simulink model "sampleModel1767_4_sub_sub_sub"  (R2023a)
settings: Solver=VariableStepAuto  StartTime=0.0  StopTime=10.0  RelTol=1e-3
libraries: simulink x5, hdlsllib x3
settings Model: Creator=user1  LastModifiedBy=user1

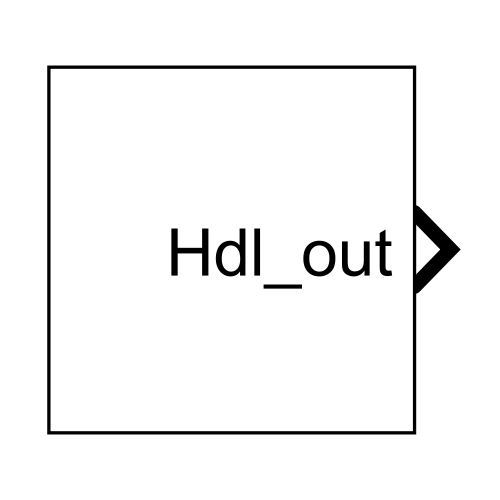
[thumbnail: Simulink's stored preview of the top-level diagram]
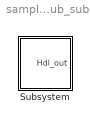
== system sampleModel1767_4_sub_sub_sub ==
  Subsystem : Subsystem

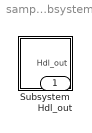
== system sampleModel1767_4_sub_sub_sub/Subsystem ==
  Subsystem : Subsystem
  Hdl_out : Outport  OutDataTypeStr=uint8

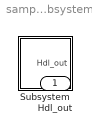
== system sampleModel1767_4_sub_sub_sub/Subsystem/Subsystem ==
  Subsystem : Subsystem
  Hdl_out : Outport  OutDataTypeStr=uint8

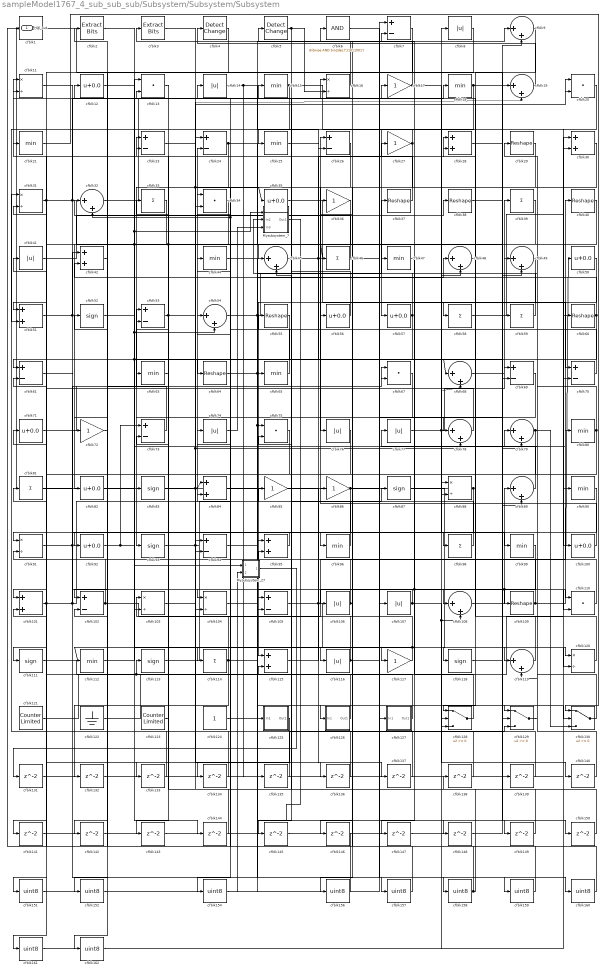
== system sampleModel1767_4_sub_sub_sub/Subsystem/Subsystem/Subsystem ==
  Mysubsystem_27 : Subsystem  TreatAsAtomicUnit=on  RTWFcnName=Mysubsystem_27
      settings: RTWFcnNameOpts=User specified  RTWFileNameOpts=Use function name
  Mysubsystem_7 : Subsystem  TreatAsAtomicUnit=on  RTWFcnName=Mysubsystem_7
      settings: RTWFcnNameOpts=User specified  RTWFileNameOpts=Use function name
  cfblk1 : hdlsllib/Logic and Bit Operations/Compare To Constant  relop=<=  const=3.0  OutDataTypeStr=uint8
  cfblk{12,35,50,56..57,71,82,92,100} (9 alike) : Bias  Bias=0.0  SaturateOnIntegerOverflow=off
  cfblk{28,30,42,51,84,95,101,115} (8 alike) : Sum  OutDataTypeStr=uint8
  cfblk{7,23..24,26,53,61,69..70,73,94,102,105} (12 alike) : Sum  Inputs=+-  OutDataTypeStr=uint8
  cfblk{11,16,31,88,91,103..104,120} (8 alike) : Product  Inputs=*/  OutDataTypeStr=uint8  RndMeth=Zero  SaturateOnIntegerOverflow=on
  cfblk{8,14,41,74,76..77,106..107,116} (9 alike) : Abs  OutDataTypeStr=uint8  SaturateOnIntegerOverflow=off
  cfblk{9,19,32,45,48..49,54,68,78..79,89,108,119} (13 alike) : Sum  Inputs=|++  OutDataTypeStr=uint8
  cfblk{29,37..38,40,55,60,64,109} (8 alike) : Reshape
  cfblk{13,20,34,67,75,110} (6 alike) : DotProduct  OutDataTypeStr=uint8
  cfblk{52,83,87,93,111,113,118} (7 alike) : Signum
  cfblk{15,18,21,25,44,47,63,65,80,90,96,99,112} (13 alike) : MinMax  OutDataTypeStr=uint8
  cfblk{33,39,46,58..59,81,98,114} (8 alike) : Sum  Inputs=+  OutDataTypeStr=uint8
  cfblk{17,27,36,72,85..86,117} (7 alike) : Gain  OutDataTypeStr=uint8
  cfblk121 : hdlsllib/Sources/Counter Limited  uplimit=7  tsamp=-1
  cfblk122 : Ground
  cfblk123 : hdlsllib/Sources/Counter Limited  uplimit=7  tsamp=-1
  cfblk124 : Constant  OutDataTypeStr=uint8  SampleTime=-1
  cfblk125 : Subsystem
      settings: LibrarySourceBlock=|
      | hdlsllib/Ports &
      | Subsystems/Subsystem
  cfblk126 : Subsystem
      settings: LibrarySourceBlock=|
      | hdlsllib/Ports &
      | Subsystems/Subsystem
  cfblk127 : Subsystem
      settings: LibrarySourceBlock=|
      | hdlsllib/Ports &
      | Subsystems/Subsystem
  cfblk128 : Switch  OutDataTypeStr=uint8  SaturateOnIntegerOverflow=off  InputSameDT=off
  cfblk129 : Switch  OutDataTypeStr=uint8  SaturateOnIntegerOverflow=off  InputSameDT=off
  cfblk130 : Switch  OutDataTypeStr=uint8  SaturateOnIntegerOverflow=off  InputSameDT=off
  cfblk{131..150} (20 alike) : Delay  SampleTime=1
  cfblk{151..152,154,156..162} (10 alike) : DataTypeConversion  OutDataTypeStr=uint8  SaturateOnIntegerOverflow=off  RndMeth=Floor
  cfblk2 : simulink/Logic and Bit Operations/Extract Bits  bitsToExtract=Upper half  numBits=8  bitIdxRange=[0 7]  outScalingMode=Preserve fixed-point scaling
      settings: LibrarySourceBlock=|
      | hdlsllib/Logic and Bit
      | Operations/Extract Bits
  cfblk3 : simulink/Logic and Bit Operations/Extract Bits  bitsToExtract=Upper half  numBits=8  bitIdxRange=[0 7]  outScalingMode=Preserve fixed-point scaling
      settings: LibrarySourceBlock=|
      | hdlsllib/Logic and Bit
      | Operations/Extract Bits
  cfblk4 : simulink/Logic and Bit Operations/Detect Change  vinit=0  OutDataTypeStr=uint8
      settings: LibrarySourceBlock=|
      | hdlsllib/Logic and Bit
      | Operations/Detect
      | Change
  cfblk5 : simulink/Logic and Bit Operations/Detect Change  vinit=0  OutDataTypeStr=uint8
      settings: LibrarySourceBlock=|
      | hdlsllib/Logic and Bit
      | Operations/Detect
      | Change
  cfblk6 : simulink/Logic and Bit Operations/Bitwise Operator  logicop=AND  UseBitMask=on  BitMask=bin2dec('11011001')  BitMaskRealWorld=Stored Integer
      settings: LibrarySourceBlock=|
      | hdlsllib/Logic and Bit
      | Operations/Bitwise
      | Operator
  Hdl_out : Outport  OutDataTypeStr=uint8
  wires:
  cfblk32/1 -> cfblk14/1
  cfblk31/1 -> cfblk61/1, cfblk18/1, cfblk45/1
  cfblk99/1 -> cfblk147/1, cfblk146/1
  cfblk33/1 -> cfblk82/1
  cfblk101/1 -> cfblk41/1, cfblk67/1, cfblk24/2
  cfblk65/1 -> cfblk34/1
  cfblk67/1 -> cfblk93/1
  cfblk21/1 -> cfblk130/1
  cfblk7/1 -> cfblk102/1
  cfblk102/1 -> cfblk71/1, cfblk40/1
  cfblk41/1 -> cfblk38/1
  cfblk119/1 -> cfblk12/1
  cfblk109/1 -> cfblk31/2, cfblk50/1
  cfblk108/1 -> cfblk89/1
  cfblk73/1 -> cfblk52/1
  cfblk55/1 -> cfblk115/1
  cfblk92/1 -> cfblk73/1, cfblk80/1
  cfblk6/1 -> cfblk158/1
  cfblk59/1 -> cfblk15/1
  cfblk29/1 -> cfblk83/1
  cfblk9/1 -> cfblk128/1
  cfblk11/1 -> cfblk96/1
  cfblk49/1 -> cfblk65/1
  cfblk80/1 -> cfblk49/1, cfblk91/1
  cfblk98/1 -> cfblk26/1
  cfblk71/1 -> cfblk53/1
  cfblk19/1 -> cfblk4/1
  cfblk68/1 -> cfblk39/1
  cfblk57/1 -> cfblk111/1, Mysubsystem_7/2(In2)
  cfblk40/1 -> cfblk76/1
  cfblk30/1 -> cfblk56/1
  cfblk113/1 -> cfblk85/1
  cfblk17/1 -> cfblk79/2, cfblk5/1
  cfblk34/1 -> cfblk143/1, cfblk72/1
  cfblk111/1 -> cfblk115/2
  cfblk95/1 -> cfblk92/1
  cfblk112/1 -> cfblk13/1
  cfblk46/1 -> cfblk78/1, cfblk32/1
  cfblk18/1 -> cfblk89/2, cfblk57/1
  cfblk93/1 -> cfblk110/1, cfblk19/2, cfblk87/1
  cfblk87/1 -> cfblk120/1
  cfblk122/1 -> cfblk8/1
  cfblk100/1 -> cfblk86/1
  cfblk86/1 -> cfblk103/2, cfblk129/1
  cfblk35/1 -> cfblk70/1
  cfblk79/1 -> cfblk130/3, cfblk95/1
  cfblk47/1 -> cfblk117/1
  cfblk61/1 -> cfblk98/1
  cfblk27/1 -> cfblk25/1, cfblk116/1
  cfblk54/1 -> cfblk130/2, cfblk48/1, cfblk37/1
  cfblk106/1 -> cfblk156/1, cfblk55/1
  cfblk45/1 -> cfblk27/1, cfblk88/2
  cfblk83/1 -> cfblk84/1, cfblk20/1, cfblk78/2
  cfblk39/1 -> cfblk64/1
  cfblk64/1 -> cfblk148/1, cfblk47/1
  cfblk115/1 -> cfblk28/1
  cfblk128/1 -> cfblk7/2
  cfblk105/1 -> cfblk79/1, cfblk127/1(In1)
  cfblk126/1(Out1) -> cfblk61/2, cfblk113/1
  cfblk16/1 -> cfblk3/1
  cfblk89/1 -> cfblk17/1
  cfblk70/1 -> cfblk32/2, cfblk13/2
  cfblk15/1 -> cfblk51/2, cfblk100/1
  cfblk37/1 -> cfblk11/1
  cfblk77/1 -> cfblk99/1, cfblk69/1
  cfblk84/1 -> cfblk110/2, cfblk109/1
  cfblk14/1 -> cfblk135/1, cfblk26/2
  cfblk50/1 -> cfblk58/1
  cfblk53/1 -> cfblk33/1, cfblk120/2
  cfblk118/1 -> cfblk19/1
  cfblk107/1 -> cfblk140/1, cfblk106/1
  cfblk120/1 -> cfblk28/2
  cfblk58/1 -> cfblk30/2
  cfblk94/1 -> cfblk9/1, cfblk75/1
  cfblk91/1 -> cfblk157/1, cfblk67/2
  cfblk48/1 -> cfblk108/1
  cfblk82/1 -> cfblk16/1, Mysubsystem_7/1(In1)
  cfblk5/1 -> cfblk16/2, cfblk105/1
  cfblk76/1 -> cfblk114/1
  cfblk90/1 -> cfblk161/1
  cfblk12/1 -> cfblk46/1, cfblk54/2, cfblk118/1, cfblk68/1
  cfblk110/1 -> cfblk36/1
  cfblk88/1 -> Hdl_out/1, cfblk101/1
  cfblk23/1 -> cfblk119/1, cfblk35/1
  cfblk121/1 -> cfblk60/1
  cfblk51/1 -> cfblk160/1, cfblk42/1
  cfblk114/1 -> cfblk132/1, cfblk20/2, cfblk23/2
  cfblk127/1(Out1) -> cfblk103/1
  cfblk123/1 -> cfblk23/1
  cfblk117/1 -> cfblk112/1, cfblk95/2
  cfblk20/1 -> cfblk70/2
  cfblk56/1 -> cfblk11/2
  cfblk24/1 -> cfblk49/2, cfblk94/2
  cfblk130/1 -> cfblk77/1
  cfblk81/1 -> cfblk104/1
  cfblk8/1 -> cfblk51/1
  cfblk78/1 -> cfblk21/1
  cfblk124/1 -> cfblk105/2
  cfblk25/1 -> cfblk69/2
  cfblk13/1 -> cfblk63/1
  cfblk129/1 -> cfblk29/1
  cfblk1/1 -> cfblk59/1
  cfblk60/1 -> cfblk42/2, cfblk104/2
  cfblk104/1 -> cfblk126/1(In1)
  cfblk96/1 -> cfblk75/2
  cfblk3/1 -> cfblk34/2
  cfblk116/1 -> cfblk73/2, cfblk128/3
  cfblk131/1 -> cfblk30/1
  cfblk132/1 -> cfblk94/1
  cfblk63/1 -> cfblk133/1
  cfblk133/1 -> cfblk31/1
  cfblk26/1 -> cfblk134/1
  cfblk134/1 -> cfblk101/2
  cfblk135/1 -> cfblk129/3
  cfblk103/1 -> cfblk136/1
  cfblk136/1 -> cfblk54/1
  cfblk85/1 -> cfblk137/1
  cfblk137/1 -> cfblk84/2
  cfblk138/1 -> cfblk91/2
  cfblk28/1 -> cfblk139/1
  cfblk139/1 -> cfblk88/1
  cfblk140/1 -> cfblk119/2
  cfblk36/1 -> cfblk141/1
  cfblk141/1 -> cfblk128/2
  cfblk72/1 -> cfblk142/1
  cfblk142/1 -> cfblk102/2
  cfblk143/1 -> cfblk9/2
  cfblk52/1 -> cfblk144/1
  cfblk144/1 -> cfblk24/1
  cfblk69/1 -> cfblk145/1
  cfblk145/1 -> cfblk7/1
  cfblk146/1 -> cfblk1/1
  cfblk147/1 -> cfblk48/2
  cfblk148/1 -> cfblk129/2
  cfblk149/1 -> cfblk53/2
  cfblk38/1 -> cfblk150/1
  cfblk150/1 -> cfblk45/2
  cfblk125/1(Out1) -> cfblk151/1
  cfblk151/1 -> cfblk107/1
  cfblk4/1 -> cfblk152/1
  cfblk152/1 -> cfblk125/1(In1)
  cfblk75/1 -> cfblk154/1
  cfblk156/1 -> cfblk2/1
  cfblk157/1 -> cfblk6/1
  cfblk158/1 -> cfblk81/1, cfblk138/1
  cfblk44/1 -> cfblk159/1
  cfblk159/1 -> cfblk74/1
  cfblk160/1 -> cfblk44/1
  cfblk161/1 -> cfblk108/2, cfblk68/2
  cfblk42/1 -> cfblk162/1
  cfblk162/1 -> cfblk90/1
  cfblk74/1 -> Mysubsystem_7/3(In3)
  Mysubsystem_7/1(Out1) -> cfblk149/1
  cfblk2/1 -> Mysubsystem_27/1(In1)
  cfblk154/1 -> Mysubsystem_27/2(In2)
  Mysubsystem_27/1(Out1) -> cfblk131/1

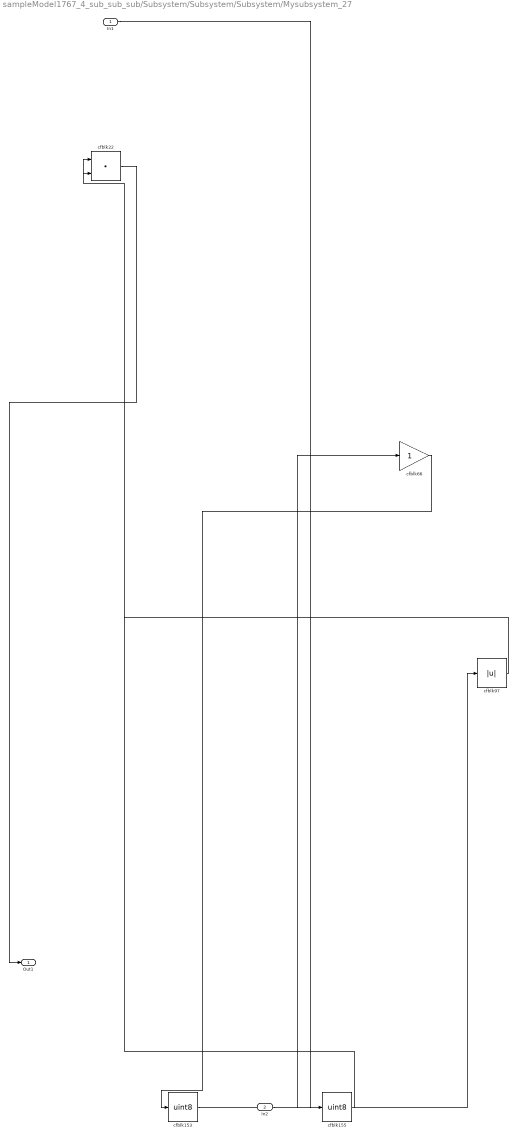
== system sampleModel1767_4_sub_sub_sub/Subsystem/Subsystem/Subsystem/Mysubsystem_27 ==
  In1 : Inport
  In2 : Inport  Port=2
  cfblk153 : DataTypeConversion  OutDataTypeStr=uint8  SaturateOnIntegerOverflow=off  RndMeth=Floor
  cfblk155 : DataTypeConversion  OutDataTypeStr=uint8  SaturateOnIntegerOverflow=off  RndMeth=Floor
  cfblk22 : DotProduct  OutDataTypeStr=Inherit: Inherit via internal rule
  cfblk66 : Gain
  cfblk97 : Abs  SaturateOnIntegerOverflow=off
  Out1 : Outport
  wires:
  cfblk22/1 -> Out1/1
  cfblk66/1 -> cfblk153/1
  cfblk155/1 -> cfblk22/2
  cfblk153/1 -> cfblk97/1
  cfblk97/1 -> cfblk22/1
  In2/1 -> cfblk66/1
  In1/1 -> cfblk155/1

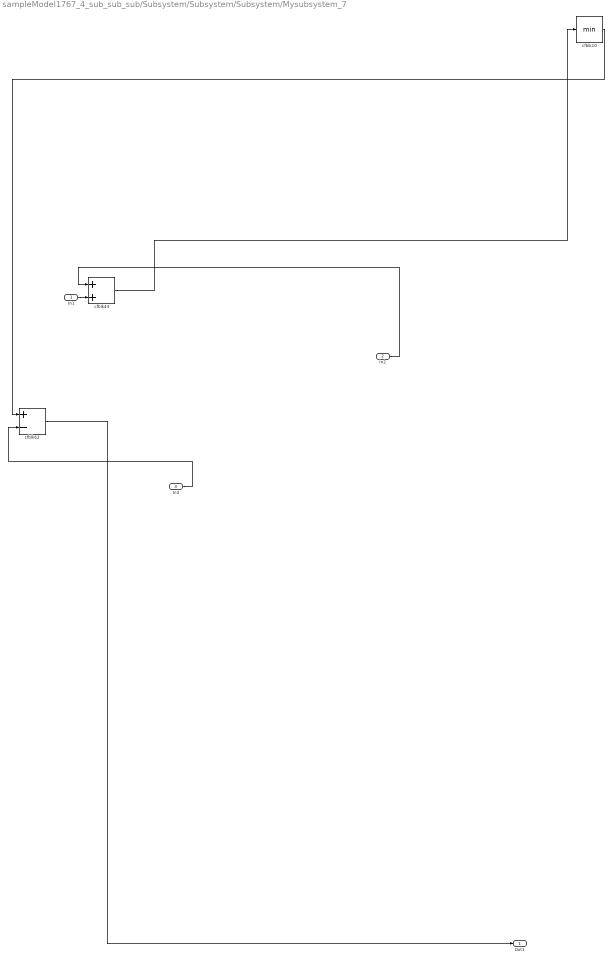
== system sampleModel1767_4_sub_sub_sub/Subsystem/Subsystem/Subsystem/Mysubsystem_7 ==
  In1 : Inport
  In2 : Inport  Port=2
  In3 : Inport  Port=3
  cfblk10 : MinMax
  cfblk43 : Sum
  cfblk62 : Sum  Inputs=+-
  Out1 : Outport
  wires:
  In2/1 -> cfblk43/1
  cfblk10/1 -> cfblk62/1
  In1/1 -> cfblk43/2
  cfblk43/1 -> cfblk10/1
  cfblk62/1 -> Out1/1
  In3/1 -> cfblk62/2

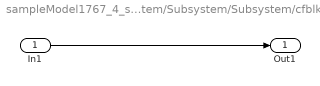
== system sampleModel1767_4_sub_sub_sub/Subsystem/Subsystem/Subsystem/cfblk125 ==
  In1 : Inport
  Out1 : Outport
  wires:
  In1/1 -> Out1/1

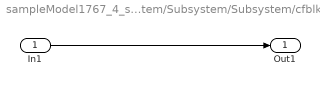
== system sampleModel1767_4_sub_sub_sub/Subsystem/Subsystem/Subsystem/cfblk126 ==
  In1 : Inport
  Out1 : Outport
  wires:
  In1/1 -> Out1/1

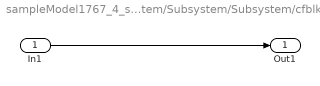
== system sampleModel1767_4_sub_sub_sub/Subsystem/Subsystem/Subsystem/cfblk127 ==
  In1 : Inport
  Out1 : Outport
  wires:
  In1/1 -> Out1/1
